simulink model "time_fuel_opt_control_of_simple_car"  (R2023b)
settings: Solver=VariableStepAuto  StartTime=0.0  StopTime=150  MaxStep=1e-4  MinStep=1e-5  RelTol=1e-3
settings Model: Creator=91798  LastModifiedBy=91798

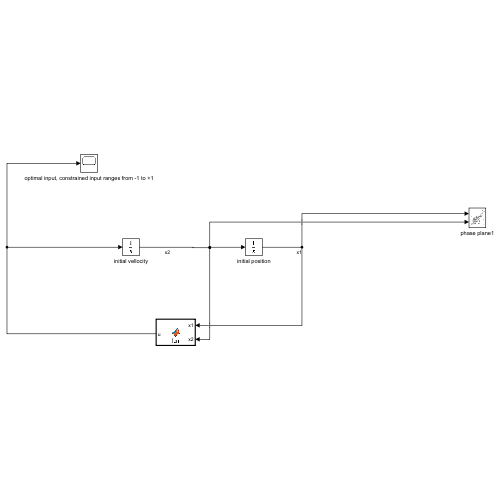
[thumbnail: Simulink's stored preview of the top-level diagram]
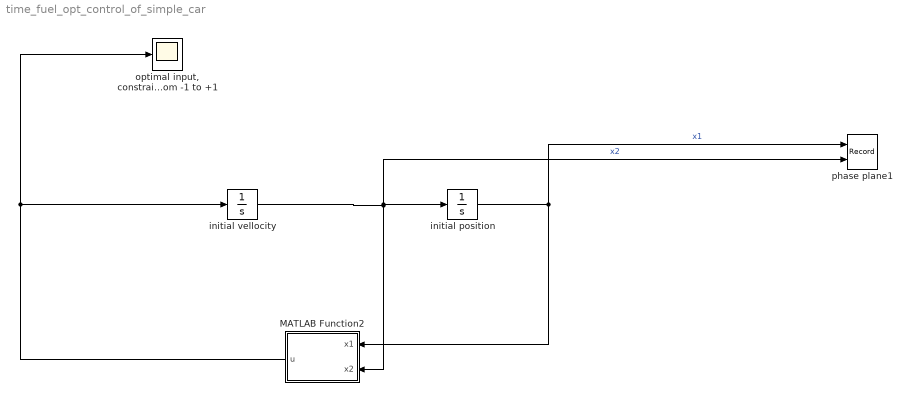
== system time_fuel_opt_control_of_simple_car ==
  MATLAB Function2 : MATLAB Function  TreatAsAtomicUnit=on
  initial position : Integrator  InitialCondition=400
  initial vellocity : Integrator  InitialCondition=6
  "optimal input, constrained input ranges from -1 to +1" : Scope
  phase plane1 : Record  FileSettingsInternal="{\"entries\":[{\"content\":{\"excelSettings\":{\"content\":{},\"type\":\"Streamout.ExcelSettings\"}},\"type\":\"Streamout.FileSettingStorage\",\"uuid\":\"\"}],\"packageUris\":[\"http:\\/\\/schema.mathworks.com\\/mf0\\/streamout_blocks\\/R2020a\"],\"version\":\"1.0\"}"  Layout=[1 1]  SignalsInternal="{\"entries\":[{\"content\":{\"signals\":[{\"content\":{\"blockPath\":[],\"dimensions\":[1],\"domain\":\"\",\"lineColor\":\"#77ac30\",\"plots\":[1],\"port\":1,\"sid\":[\"\"],\"signalID\":28976,\"signalName\":\"x1\"},\"type\":\"RecordBlkView.Signal\",\"uuid\":\"\"},{\"content\":{\"blockPath\":[],\"dimensions\":[1],\"domain\":\"\",\"lineColor\":\"#4dbeee\",\"plots\":[1],\"port\":2,\"sid\":[\"\"],\"signalID\":28980,\"signalName\":\"x2\"},\"type\":\"RecordBlkView.Signal\",\"uuid\":\"\"}]},\"type\":\"RecordBlkView.InputSignals\",\"uuid\":\"\"}],\"packageUris\":[\"http:\\/\\/schema.mathworks.com\\/mf0\\/streamout_blocks\\/R2020a\"],\"version\":\"1.0\"}"  VisualizationBindings="{\"xyplotplugin\":{\"info\":[{\"series\":[{\"bindingParametersList\":[{\"parameter\":\"X-Axis\",\"signalID\":28976,\"signalName\":\"x1\"},{\"parameter\":\"Y-Axis\",\"signalID\":28980,\"signalName\":\"x2\"}],\"seriesID\":58968}],\"subplotID\":1}]}}"  CompatibilityTag=XY  st=-1
  wires:
  MATLAB Function2/1(u) -> initial vellocity/1, "optimal input, constrained input ranges from -1 to +1"/1
  initial position/1 -> phase plane1/1, MATLAB Function2/1(x1)  "x1"
  initial vellocity/1 -> MATLAB Function2/2(x2), initial position/1, phase plane1/2  "x2"

== matlab function time_fuel_opt_control_of_simple_car/MATLAB Function2 ==
  data: x1 input; u output; x2 input
function u = fcn(x1,x2)

% cost function=integral of (k+mod(u)) from 0 to tf(final time) 
% increase k for faster reaching 0,0

k=.4/3;%user defined epsilon fuel optimal parameter, lesser it is,the lesser fuel req to reach 0,0

z=x1+0.5*x2*abs(x2);

y=  +sqrt(k*(k+2))*(2/(k+4))*x1    +  x2*sqrt(((x2^2)/2)+abs(x1));

%switching logic

if z>0 && y>0
    u=-1;
elseif ( z<0 && y<0)
    u=1;
    
else u=0;
 
  end
end
